simulink model "ABS"  (R2018b)
settings: Solver=ode45  StartTime=0.0  StopTime=10  RelTol=1e-6
settings Model: Creator=jinwooro  LastModifiedBy=jinwooro

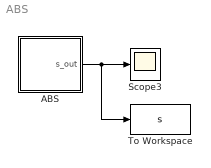
== system ABS ==
  ABS : Stateflow chart  TreatAsAtomicUnit=on
  Scope3 : Scope
  To Workspace : ToWorkspace  VariableName=s  SaveFormat=Timeseries  SampleTime=-1
  wires:
  ABS/1(s_out) -> To Workspace/1, Scope3/1

== stateflow chart ABS/ABS ==
  settings: updateMethod=CONTINUOUS
  state Lock
    du:
    s_dot = 0.13;
    s_out = s;
  state Release
    du:
    s_dot = -0.13;
    s_out = s;
  (default) -> Lock : {s = 0;}
  Lock -> Release : [s >= 0.22]
  Release -> Lock : [ s <= 0.18]
  data: s local; s_out output
  data s settings: updateMethod=SF_CONTINUOUS_TIME_DATA
